simulink model "Inverter_circuit_redesign_from_NITW_Paper23"  (R2021b)
settings: Solver=ode23t  StartTime=0.0  StopTime=2  RelTol=1e-3
values from neighbouring files (symbols this model uses):
  B = 5    [FOC_parameters_Basil.m]    (also in parameters_FOC.m = 53)
  C_LCL = 100e-6    (= 0.0001)    [FOC_parameters_Basil.m]
  D = 0.25    [FOC_parameters_Basil.m]    (also in parameters_FOC.m)
  k = 1    [FOC_parameters_Basil.m]
  L_LCL = 500e-6    (= 0.0005)    [FOC_parameters_Basil.m]
  Ll = 0.0416    [FOC_parameters_Basil.m]
  Lm = 0.0416    [FOC_parameters_Basil.m]    (also in parameters_FOC.m = 0.4)
  Lp = 0.0684    [FOC_parameters_Basil.m]
  M = 4.775    [FOC_parameters_Basil.m]    (also in parameters_FOC.m)
  P = 2    [FOC_parameters_Basil.m]    (also in parameters_FOC.m = 4)
  Rl = 0.976    [FOC_parameters_Basil.m]
  Rp = 1.298    [FOC_parameters_Basil.m]
  Tp = 0.027    [FOC_parameters_Basil.m]    (also in parameters_FOC.m = 0.0465)
  VDC = 800    [FOC_parameters_Basil.m]
undefined symbols (not defined in the file or in its folder): L
libraries: spsSeriesRLCBranchLib x9, slpidlib x6, spsIGBTDiodeLib x6, eeTransforms x4, spsCurrentMeasurementLib x3, simulink_extras x1, spsDCVoltageSourceLib x1, simulink x1, spsThreePhaseVIMeasurementLib x1, spsdq0toabcLib x1, spspowerguiLib x1
(part 2 of 2)

== matlab function Inverter_circuit_redesign_from_NITW_Paper23/Subsystem3/MATLAB Function ==
  data: f input; multiplier output; ve input; Lp input; Ll input; Lm input; Tp input
function multiplier = multiplier_calculation(f, ve, Lp, Ll, Lm, Tp)

    L_sigma = Lp - Lm*f - (Lm * (1-f))^2/(Ll - Lm*f);

    multiplier = pi*ve*L_sigma/Tp;

end
